simulink model "torqueBalancingPHRIStandup"  (Simulink 9.1)
settings: Solver=FixedStepDiscrete  StartTime=0.0  StopTime="Config.SIMULATION_TIME "  FixedStep=Config.Ts  RelTol=1e-3  EnableMultiTasking=on
InitFcn:
  | cd(fileparts(which(bdroot)));
  | initTorqueBalancingPHRIStandup;
StopFcn:
  | cd(fileparts(which(bdroot)));
  | stopTorqueBalancingPHRIStandup;
undefined symbols (not defined in the file or in its folder): bVectorConstraintsFeet, bVectorConstraintsLegs, Config, ConstraintsMatrixFeet, ConstraintsMatrixLegs, Gain, HUMAN_DOF_FOR_SIMULINK, Reg, ROBOT_DOF, ROBOT_DOF_FOR_SIMULINK, Sat, Sm
libraries: WBToolboxLibrary x153, simulink x4
(part 1 of 4)
settings Model: SuppressorTable=22 serialization::archive 11 0 6 0 0 0 1 0  Creator=daniele  LastModifiedBy=yeshi  NumberOfSteps=100
settings DataIOCC: LimitDataPoints=on
settings OptimizationCC: ExpressionDepthLimit=2147483647
settings DebuggingCC: SolverPrmCheckMsg=warning  FcnCallInpInsideContextMsg=warning  AllowSymbolicDim=off  StateNameClashWarn=warning
settings SFSimCC: SimParseCustomCode=off
settings GRTTargetCC: GeneratePreprocessorConditionals=Disable all

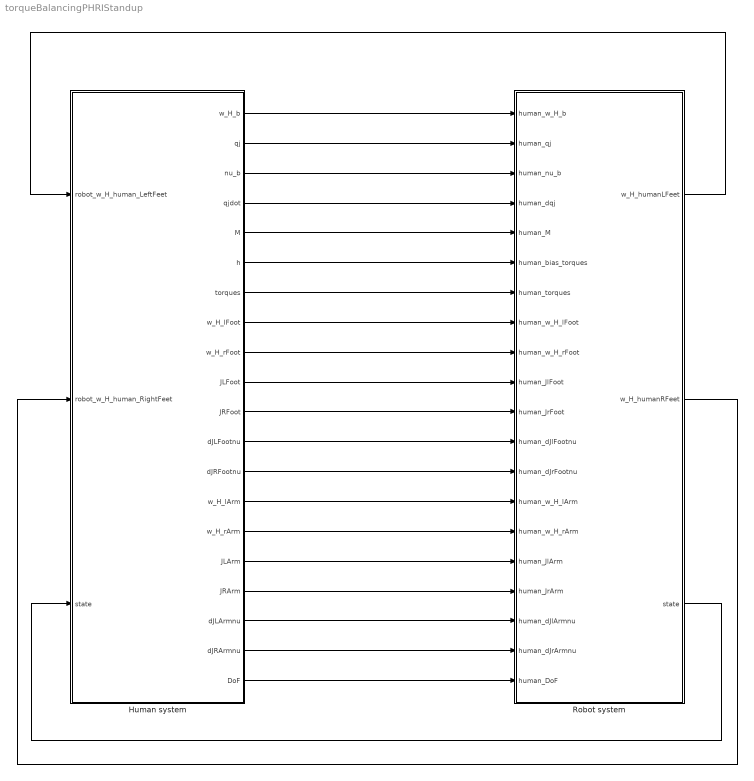
== system torqueBalancingPHRIStandup ==
  Human system : Subsystem
  Robot system : Subsystem
  wires:
  Human system/1(w_H_b) -> Robot system/1("human_w_H_b ")
  Human system/2(qj) -> Robot system/2("human_qj ")
  Human system/3(nu_b) -> Robot system/3(human_nu_b)
  Human system/4(qjdot) -> Robot system/4(human_dqj)
  Human system/5(M) -> Robot system/5(human_M)
  Human system/6(h) -> Robot system/6(human_bias_torques)
  Human system/7(torques) -> Robot system/7(human_torques)
  Human system/8(w_H_lFoot) -> Robot system/8(human_w_H_lFoot)
  Human system/9(w_H_rFoot) -> Robot system/9(human_w_H_rFoot)
  Human system/10(JLFoot) -> Robot system/10(human_JlFoot)
  Human system/11(JRFoot) -> Robot system/11(human_JrFoot)
  Human system/12(dJLFootnu) -> Robot system/12(human_dJlFootnu)
  Human system/13(dJRFootnu) -> Robot system/13(human_dJrFootnu)
  Human system/14(w_H_lArm) -> Robot system/14(human_w_H_lArm)
  Human system/15(w_H_rArm) -> Robot system/15(human_w_H_rArm)
  Human system/16(JLArm) -> Robot system/16(human_JlArm)
  Human system/17(JRArm) -> Robot system/17(human_JrArm)
  Human system/18(dJLArmnu) -> Robot system/18(human_dJlArmnu)
  Human system/19(dJRArmnu) -> Robot system/19(human_dJrArmnu)
  Human system/20(DoF) -> Robot system/20(human_DoF)
  Robot system/1(w_H_humanLFeet) -> Human system/1(robot_w_H_human_LeftFeet)
  Robot system/2(w_H_humanRFeet) -> Human system/2(robot_w_H_human_RightFeet)
  Robot system/3(state) -> Human system/3("state ")

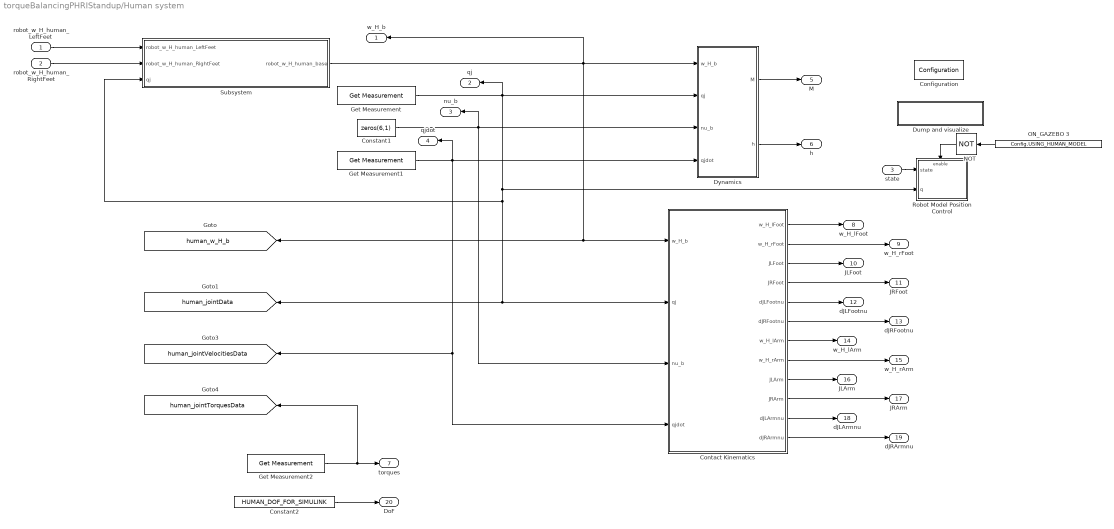
== system torqueBalancingPHRIStandup/Human system ==
  robot_w_H_human_LeftFeet : Inport
  robot_w_H_human_RightFeet : Inport  Port=2
  "state " : Inport  Port=3
  Configuration : WBToolboxLibrary/Utilities/Configuration  ConfigSource=Workspace  ConfigObject='HUMAN_WBTConfigRobot'  RobotName='icubSim'  UrdfFile='model.urdf'  ControlledJoints={'l_elbow','l_shoulder_pitch','torso_roll'}  ControlBoardsNames={'left_arm','right_arm','torso'}  LocalName='WBT'  GravityVector=[0,0,-9.81]
      settings: SourceProductName=Whole Body Toolbox
  Constant1 : Constant  Value=zeros(6,1)
  Constant2 : Constant  Value=HUMAN_DOF_FOR_SIMULINK
  Contact Kinematics : Subsystem
  Dump and visualize : Subsystem
      mask Display: disp('VISUALIZER')
  Dynamics : Subsystem
  Get Measurement : WBToolboxLibrary/wholeBodyStates/Get Measurement  measuredType=Joints Position
      settings: SourceProductName=Whole Body Toolbox
  Get Measurement1 : WBToolboxLibrary/wholeBodyStates/Get Measurement  measuredType=Joints Velocity
      settings: SourceProductName=Whole Body Toolbox
  Get Measurement2 : WBToolboxLibrary/wholeBodyStates/Get Measurement  measuredType=Joints Torque
      settings: SourceProductName=Whole Body Toolbox
  NOT : Logic  Operator=NOT  IconShape=distinctive  AllPortsSameDT=off  OutDataTypeStr=boolean
  ON_GAZEBO 3 : Constant  Value=Config.USING_HUMAN_MODEL
  Robot Model Position Control : Subsystem
  Subsystem : Subsystem
  w_H_b : Outport
  qj : Outport  Port=2
  nu_b : Outport  Port=3
  qjdot : Outport  Port=4
  M : Outport  Port=5
  h : Outport  Port=6
  torques : Outport  Port=7
  w_H_lFoot : Outport  Port=8
  w_H_rFoot : Outport  Port=9
  JLFoot : Outport  Port=10
  JRFoot : Outport  Port=11
  dJLFootnu : Outport  Port=12
  dJRFootnu : Outport  Port=13
  w_H_lArm : Outport  Port=14
  w_H_rArm : Outport  Port=15
  JLArm : Outport  Port=16
  JRArm : Outport  Port=17
  dJLArmnu : Outport  Port=18
  dJRArmnu : Outport  Port=19
  DoF : Outport  Port=20
  tag scope: human_jointData=global, human_jointTorquesData=global, human_jointVelocitiesData=global, human_w_H_b=global
  wires:
  Constant1/1 -> nu_b/1, Contact Kinematics/3(nu_b), Dynamics/3(nu_b)
  Get Measurement1/1 -> qjdot/1, Dynamics/4(qjdot), [human_jointVelocitiesData], Contact Kinematics/4(qjdot)
  Dynamics/1(M) -> M/1
  Dynamics/2(h) -> h/1
  Get Measurement2/1 -> [human_jointTorquesData], torques/1
  Contact Kinematics/1(w_H_lFoot) -> w_H_lFoot/1
  Contact Kinematics/2(w_H_rFoot) -> w_H_rFoot/1
  Contact Kinematics/3(JLFoot) -> JLFoot/1
  Contact Kinematics/4(JRFoot) -> JRFoot/1
  Contact Kinematics/5(dJLFootnu) -> dJLFootnu/1
  Contact Kinematics/6(dJRFootnu) -> dJRFootnu/1
  Contact Kinematics/7(w_H_lArm) -> w_H_lArm/1
  Contact Kinematics/8(w_H_rArm) -> w_H_rArm/1
  Contact Kinematics/9(JLArm) -> JLArm/1
  Contact Kinematics/10(JRArm) -> JRArm/1
  Contact Kinematics/11(dJLArmnu) -> dJLArmnu/1
  Contact Kinematics/12(dJRArmnu) -> dJRArmnu/1
  Constant2/1 -> DoF/1
  Get Measurement/1 -> qj/1, [human_jointData], Contact Kinematics/2(qj), Subsystem/3(qj), Robot Model Position Control/2(q), Dynamics/2(qj)
  Subsystem/1(robot_w_H_human_base) -> w_H_b/1, Contact Kinematics/1(w_H_b), [human_w_H_b], Dynamics/1(w_H_b)
  robot_w_H_human_LeftFeet/1 -> Subsystem/1(robot_w_H_human_LeftFeet)
  robot_w_H_human_RightFeet/1 -> Subsystem/2(robot_w_H_human_RightFeet)
  "state "/1 -> Robot Model Position Control/1(state)
  ON_GAZEBO 3/1 -> NOT/1
  NOT/1 -> Robot Model Position Control/Enable

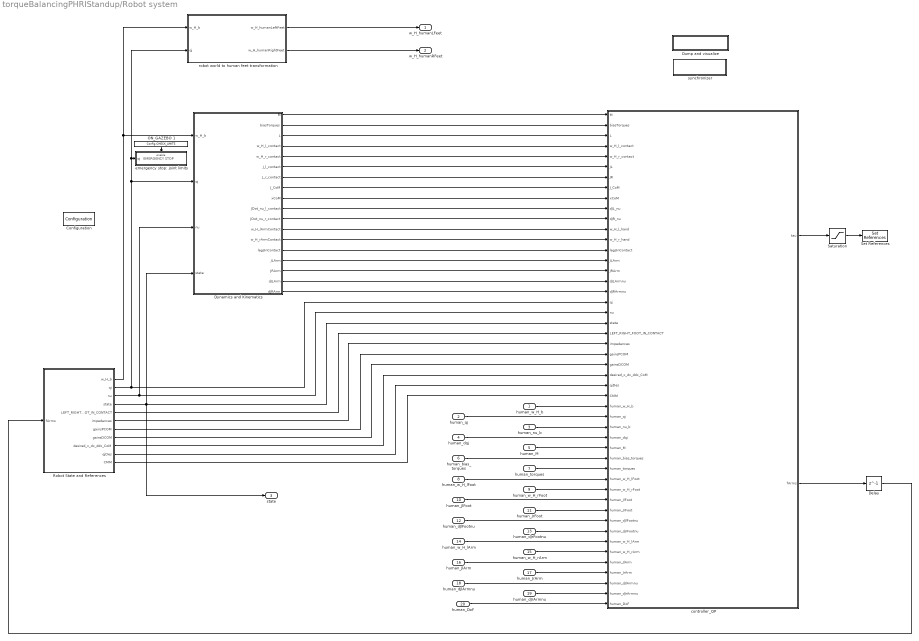
== system torqueBalancingPHRIStandup/Robot system ==
  "human_w_H_b " : Inport
  "human_qj " : Inport  Port=2
  human_nu_b : Inport  Port=3
  human_dqj : Inport  Port=4
  human_M : Inport  Port=5
  human_bias_torques : Inport  Port=6
  human_torques : Inport  Port=7
  human_w_H_lFoot : Inport  Port=8
  human_w_H_rFoot : Inport  Port=9
  human_JlFoot : Inport  Port=10
  human_JrFoot : Inport  Port=11
  human_dJlFootnu : Inport  Port=12
  human_dJrFootnu : Inport  Port=13
  human_w_H_lArm : Inport  Port=14
  human_w_H_rArm : Inport  Port=15
  human_JlArm : Inport  Port=16
  human_JrArm : Inport  Port=17
  human_dJlArmnu : Inport  Port=18
  human_dJrArmnu : Inport  Port=19
  human_DoF : Inport  Port=20
  Configuration : WBToolboxLibrary/Utilities/Configuration  ConfigSource=Workspace  ConfigObject='WBTConfigRobot'  RobotName='icubSim'  UrdfFile='model.urdf'  ControlledJoints={'l_elbow','l_shoulder_pitch','torso_roll'}  ControlBoardsNames={'left_arm','right_arm','torso'}  LocalName='WBT'  GravityVector=[0,0,-9.81]
      settings: SourceProductName=Whole Body Toolbox
  Delay : Delay  DelayLength=1
  Dump and visualize : Subsystem
      mask Display: disp('VISUALIZER')
  Dynamics and Kinematics : Subsystem
  ON_GAZEBO 1 : Constant  Value=Config.CHECK_LIMITS
  Robot State and References : Subsystem  Priority=-10
  Saturation : Saturate  UpperLimit=Sat.torque  LowerLimit=-Sat.torque
  Set References : WBToolboxLibrary/wholeBodyActuators/Set References  controlType=Torque  refSpeed=50  refAcceleration=1000000*(pi/180)
      settings: SourceProductName=Whole Body Toolbox
  controller_QP : Subsystem
  emergency stop: joint limits : Subsystem
  robot world to human feet transformation : Subsystem
  synchronizer : Subsystem
      mask Display: disp('SYNCHRONIZER')
  w_H_humanLFeet : Outport
  w_H_humanRFeet : Outport  Port=2
  state : Outport  Port=3
  wires:
  Dynamics and Kinematics/9(xCoM) -> controller_QP/9(xCoM)
  Saturation/1 -> Set References/1
  Robot State and References/6(impedances) -> controller_QP/23(impedances)
  Robot State and References/7(gainsPCOM) -> controller_QP/24(gainsPCOM)
  Dynamics and Kinematics/10(JDot_nu_l_contact) -> controller_QP/10(dJL_nu)
  Robot State and References/5(LEFT_RIGHT_FOOT_IN_CONTACT) -> controller_QP/22(LEFT_RIGHT_FOOT_IN_CONTACT)
  Dynamics and Kinematics/2(biasTorques) -> controller_QP/2(biasTorques)
  ON_GAZEBO 1/1 -> emergency stop: joint limits/Enable
  Dynamics and Kinematics/6(J_l_contact) -> controller_QP/6(JL)
  Dynamics and Kinematics/14(legsInContact) -> controller_QP/14(legsInContact)
  Dynamics and Kinematics/8(J_CoM) -> controller_QP/8(J_CoM)
  Robot State and References/4(state) -> state/1, Dynamics and Kinematics/4("state "), controller_QP/21(state)
  Dynamics and Kinematics/4(w_H_l_contact) -> controller_QP/4(w_H_l_contact)
  Robot State and References/2(qj) -> robot world to human feet transformation/2(qj), emergency stop: joint limits/1(qj   EMERGENCY STOP), Dynamics and Kinematics/2(qj), controller_QP/19(qj)
  Dynamics and Kinematics/11(JDot_nu_r_contact) -> controller_QP/11(dJR_nu)
  Robot State and References/10(qjDes) -> controller_QP/27(qjDes)
  Robot State and References/9(desired_x_dx_ddx_CoM) -> controller_QP/26(desired_x_dx_ddx_CoM)
  Dynamics and Kinematics/1(M) -> controller_QP/1(M)
  Dynamics and Kinematics/5(w_H_r_contact) -> controller_QP/5(w_H_r_contact)
  Robot State and References/8(gainsDCOM) -> controller_QP/25(gainsDCOM)
  Robot State and References/1(w_H_b) -> robot world to human feet transformation/1(w_H_b), Dynamics and Kinematics/1(w_H_b)
  Robot State and References/3(nu) -> Dynamics and Kinematics/3(nu), controller_QP/20(nu)
  controller_QP/1("tau ") -> Saturation/1
  Dynamics and Kinematics/7(J_r_contact) -> controller_QP/7(JR)
  Dynamics and Kinematics/3(L) -> controller_QP/3("L ")
  robot world to human feet transformation/2(w_H_humanRightFeet) -> w_H_humanRFeet/1
  robot world to human feet transformation/1(w_H_humanLeftFeet) -> w_H_humanLFeet/1
  "human_w_H_b "/1 -> controller_QP/29("human_w_H_b ")
  "human_qj "/1 -> controller_QP/30("human_qj ")
  human_nu_b/1 -> controller_QP/31(human_nu_b)
  human_dqj/1 -> controller_QP/32(human_dqj)
  human_M/1 -> controller_QP/33(human_M)
  human_bias_torques/1 -> controller_QP/34(human_bias_torques)
  human_torques/1 -> controller_QP/35(human_torques)
  human_w_H_lFoot/1 -> controller_QP/36(human_w_H_lFoot)
  human_w_H_rFoot/1 -> controller_QP/37(human_w_H_rFoot)
  human_JlFoot/1 -> controller_QP/38(human_JlFoot)
  human_JrFoot/1 -> controller_QP/39(human_JrFoot)
  human_dJlFootnu/1 -> controller_QP/40(human_dJlFootnu)
  human_dJrFootnu/1 -> controller_QP/41(human_dJrFootnu)
  human_w_H_lArm/1 -> controller_QP/42(human_w_H_lArm)
  human_w_H_rArm/1 -> controller_QP/43(human_w_H_rArm)
  human_JlArm/1 -> controller_QP/44(human_JlArm)
  human_JrArm/1 -> controller_QP/45(human_JrArm)
  human_dJlArmnu/1 -> controller_QP/46(human_dJlArmnu)
  human_dJrArmnu/1 -> controller_QP/47(human_dJrArmnu)
  human_DoF/1 -> controller_QP/48(human_DoF)
  Dynamics and Kinematics/12(w_H_lArmContact) -> controller_QP/12(w_H_l_hand)
  Dynamics and Kinematics/13(w_H_rArmContact) -> controller_QP/13(w_H_r_hand)
  Dynamics and Kinematics/15(JLArm) -> controller_QP/15(JLArm)
  Dynamics and Kinematics/16(JRArm) -> controller_QP/16(JRArm)
  Dynamics and Kinematics/17(dJLArm) -> controller_QP/17(dJLArmnu)
  Dynamics and Kinematics/18(dJRArm) -> controller_QP/18(dJRArmnu)
  controller_QP/2(fArms) -> Delay/1
  Delay/1 -> Robot State and References/1(fArms)
  Robot State and References/11(CMM) -> controller_QP/28(CMM)

== system torqueBalancingPHRIStandup/Human system/Contact Kinematics ==
  w_H_b : Inport
  qj : Inport  Port=2
  nu_b : Inport  Port=3
  qjdot : Inport  Port=4
  Arm Contact Kinematics : Subsystem
  Leg Contact Kinematics : Subsystem
  w_H_lFoot : Outport
  w_H_rFoot : Outport  Port=2
  JLFoot : Outport  Port=3
  JRFoot : Outport  Port=4
  dJLFootnu : Outport  Port=5
  dJRFootnu : Outport  Port=6
  w_H_lArm : Outport  Port=7
  w_H_rArm : Outport  Port=8
  JLArm : Outport  Port=9
  JRArm : Outport  Port=10
  dJLArmnu : Outport  Port=11
  dJRArmnu : Outport  Port=12
  wires:
  w_H_b/1 -> Arm Contact Kinematics/1(w_H_b), Leg Contact Kinematics/1(w_H_b)
  qj/1 -> Arm Contact Kinematics/2(qj), Leg Contact Kinematics/2(qj)
  nu_b/1 -> Leg Contact Kinematics/3(nu_b), Arm Contact Kinematics/3(nu_b)
  qjdot/1 -> Arm Contact Kinematics/4(qjdot), Leg Contact Kinematics/4(qjdot)
  Leg Contact Kinematics/1(w_H_lFoot) -> w_H_lFoot/1
  Leg Contact Kinematics/2(w_H_rFoot) -> w_H_rFoot/1
  Leg Contact Kinematics/3(JLFoot) -> JLFoot/1
  Leg Contact Kinematics/4(JRFoot) -> JRFoot/1
  Leg Contact Kinematics/5(dJLFootnu) -> dJLFootnu/1
  Leg Contact Kinematics/6(dJRFootnu) -> dJRFootnu/1
  Arm Contact Kinematics/2(w_H_rArm) -> w_H_rArm/1
  Arm Contact Kinematics/1(w_H_lArm) -> w_H_lArm/1
  Arm Contact Kinematics/3(JLArm) -> JLArm/1
  Arm Contact Kinematics/5(dJLArmnu) -> dJLArmnu/1
  Arm Contact Kinematics/6(dJRArmnu) -> dJRArmnu/1
  Arm Contact Kinematics/4(JRArm) -> JRArm/1

== system torqueBalancingPHRIStandup/Human system/Dump and visualize ==
  Human data : Subsystem
  Logical Operator1 : Logic  Operator=OR  AllPortsSameDT=off  OutDataTypeStr=boolean
  ON_GAZEBO 3 : Constant  Value=Config.SCOPES_ALL
  ON_GAZEBO 4 : Constant  Value=Config.SCOPES_MAIN
  wires:
  ON_GAZEBO 3/1 -> Logical Operator1/1
  ON_GAZEBO 4/1 -> Logical Operator1/2
  Logical Operator1/1 -> Human data/Enable
  [human_jointVelocitiesData] -> Human data/3(human_jointVelocitiesData)
  [human_jointTorquesData] -> Human data/4(human_jointTorquesData)
  [human_w_H_b] -> Human data/1(human_w_H_b)
  [human_jointData] -> Human data/2(human_jointData)

== system torqueBalancingPHRIStandup/Human system/Dynamics ==
  w_H_b : Inport
  qj : Inport  Port=2
  nu_b : Inport  Port=3
  qjdot : Inport  Port=4
  Get Bias Forces : WBToolboxLibrary/wholeBodyModel/Dynamics/Get Bias Forces
      settings: SourceProductName=Whole Body Toolbox
  Mass Matrix : WBToolboxLibrary/wholeBodyModel/Dynamics/Mass Matrix
      settings: SourceProductName=Whole Body Toolbox
  M : Outport
  h : Outport  Port=2
  wires:
  qjdot/1 -> Get Bias Forces/4
  nu_b/1 -> Get Bias Forces/3
  qj/1 -> Get Bias Forces/2, Mass Matrix/2
  Get Bias Forces/1 -> h/1
  w_H_b/1 -> Get Bias Forces/1, Mass Matrix/1
  Mass Matrix/1 -> M/1

== system torqueBalancingPHRIStandup/Human system/Robot Model Position Control ==
  state : Inport
  q : Inport  Port=2
  Enable : EnablePort
  Clock : Clock
  Constant : Constant  Value=2
  Demux1 : Demux  Outputs=Config.numOfJointsForEachControlboard
  Minimum Jerk Trajectory Generator1 : WBToolboxLibrary/Utilities/Minimum Jerk Trajectory Generator  externalSettlingTime=on  settlingTime=1  sampleTime=Config.Ts  resetOnSettlingTime=off  firstDerivatives=off  secondDerivatives=off  explicitInitialValue=off
      settings: SourceProductName=Whole Body Toolbox
  Set References : WBToolboxLibrary/wholeBodyActuators/Set References  controlType=Position Direct  refSpeed=2*(pi/180)  refAcceleration=1000000*(pi/180)
      settings: SourceProductName=Whole Body Toolbox
  getJointRef : MATLAB Function  TreatAsAtomicUnit=on
  joint references : Scope  NumInputPorts=6
  wires:
  getJointRef/1(joint_ref) -> Minimum Jerk Trajectory Generator1/1
  Constant/1 -> Minimum Jerk Trajectory Generator1/2
  Demux1/3 -> joint references/3  "right_arm"
  Demux1/5 -> joint references/5  "right_leg"
  Demux1/4 -> joint references/4  "left_leg"
  Demux1/2 -> joint references/2  "left_arm"
  Minimum Jerk Trajectory Generator1/1 -> Demux1/1, Set References/1
  state/1 -> getJointRef/3(state), joint references/6
  Demux1/1 -> joint references/1  "torso"
  Clock/1 -> getJointRef/1(sim_time)
  q/1 -> getJointRef/2(q)

== system torqueBalancingPHRIStandup/Human system/Subsystem ==
  robot_w_H_human_LeftFeet : Inport
  robot_w_H_human_RightFeet : Inport  Port=2
  qj : Inport  Port=3
  Constant3 : Constant  Value=eye(4)
  Forward Kinematics : WBToolboxLibrary/wholeBodyModel/Kinematics/Forward Kinematics  frameName=HUMAN_Frames.LEFT_FOOT
      settings: SourceProductName=Whole Body Toolbox
  "Inv\\*  " : Product  Inputs=*/  Multiplication=Matrix(*)
  Switch : Switch  Criteria=u2 > Threshold
  switch threshold : Constant
  robot_w_H_human_base : Outport
  wires:
  robot_w_H_human_RightFeet/1 -> Switch/3
  "Inv\\*  "/1 -> robot_w_H_human_base/1
  qj/1 -> Forward Kinematics/2
  switch threshold/1 -> Switch/2
  Constant3/1 -> Forward Kinematics/1
  Switch/1 -> "Inv\\*  "/1
  Forward Kinematics/1 -> "Inv\\*  "/2
  robot_w_H_human_LeftFeet/1 -> Switch/1

== system torqueBalancingPHRIStandup/Robot system/Dump and visualize ==
  Human assistance : Subsystem
  Logical Operator2 : Logic  Operator=OR  AllPortsSameDT=off  OutDataTypeStr=boolean
  ON_GAZEBO 1 : Constant  Value=Config.SCOPES_ALL
  ON_GAZEBO 2 : Constant  Value=Config.SCOPES_MAIN
  Robot data1 : Subsystem
  wires:
  [alpha] -> Human assistance/2(alpha)
  [fArms] -> Human assistance/3(fArms)
  [phri_human_feet_wrench] -> Human assistance/4(phri_human_feet_wrench)
  [phri_robot_feet_wrench] -> Human assistance/5(phri_robot_feet_wrench)
  [f_noQP] -> Robot data1/8(fDesNoQP)
  ON_GAZEBO 2/1 -> Logical Operator2/2
  [CoM_error] -> Robot data1/5(CoM_Error)
  [state] -> Human assistance/1(state), Robot data1/3(state)
  [qj_des] -> Robot data1/4(qj_des)
  [CoM_des] -> Robot data1/7(CoM_des)
  [w_H_b] -> Robot data1/2(w_H_b)
  Logical Operator2/1 -> Robot data1/Enable
  ON_GAZEBO 1/1 -> Logical Operator2/1
  [tau_des] -> Robot data1/1(tau_des)
  [f_QP] -> Robot data1/6(fDesQP)

== system torqueBalancingPHRIStandup/Robot system/Dynamics and Kinematics ==
  w_H_b : Inport
  qj : Inport  Port=2
  nu : Inport  Port=3
  "state " : Inport  Port=4
  Dynamics : Subsystem
  Kinematics : Subsystem
  M : Outport
  biasTorques : Outport  Port=2
  L : Outport  Port=3
  w_H_l_contact : Outport  Port=4
  w_H_r_contact : Outport  Port=5
  J_l_contact : Outport  Port=6
  J_r_contact : Outport  Port=7
  J_CoM : Outport  Port=8
  xCoM : Outport  Port=9
  JDot_nu_l_contact : Outport  Port=10
  JDot_nu_r_contact : Outport  Port=11
  w_H_lArmContact : Outport  Port=12
  w_H_rArmContact : Outport  Port=13
  legsInContact : Outport  Port=14
  JLArm : Outport  Port=15
  JRArm : Outport  Port=16
  dJLArm : Outport  Port=17
  dJRArm : Outport  Port=18
  wires:
  w_H_b/1 -> Kinematics/3(w_H_b), Dynamics/1(w_H_b)
  qj/1 -> Dynamics/2(qj), Kinematics/2(qj)
  nu/1 -> Dynamics/3(nu), Kinematics/1(nu)
  Dynamics/1(M(q)) -> M/1
  Dynamics/2(biasTorques) -> biasTorques/1
  Dynamics/3(L(q,dq)) -> L/1
  Kinematics/5(J_CoM) -> J_CoM/1
  Kinematics/6(xCoM) -> xCoM/1
  Kinematics/1(w_H_l_contact) -> w_H_l_contact/1
  Kinematics/2(w_H_r_contact) -> w_H_r_contact/1
  Kinematics/7(JDot_nu_l_contact) -> JDot_nu_l_contact/1
  Kinematics/8(JDot_nu_r_contact) -> JDot_nu_r_contact/1
  Kinematics/3(J_l_contact) -> J_l_contact/1
  Kinematics/4(J_r_contact) -> J_r_contact/1
  Kinematics/9(legsInContact) -> legsInContact/1
  "state "/1 -> Kinematics/4("state ")
  Kinematics/12(JLArm) -> JLArm/1
  Kinematics/11(w_H_rArmContact) -> w_H_rArmContact/1
  Kinematics/13(JRArm) -> JRArm/1
  Kinematics/15(JDot_nu_rArm_contact) -> dJRArm/1
  Kinematics/14(JDot_nu_lArm_contact) -> dJLArm/1
  Kinematics/10(w_H_lArmContact) -> w_H_lArmContact/1

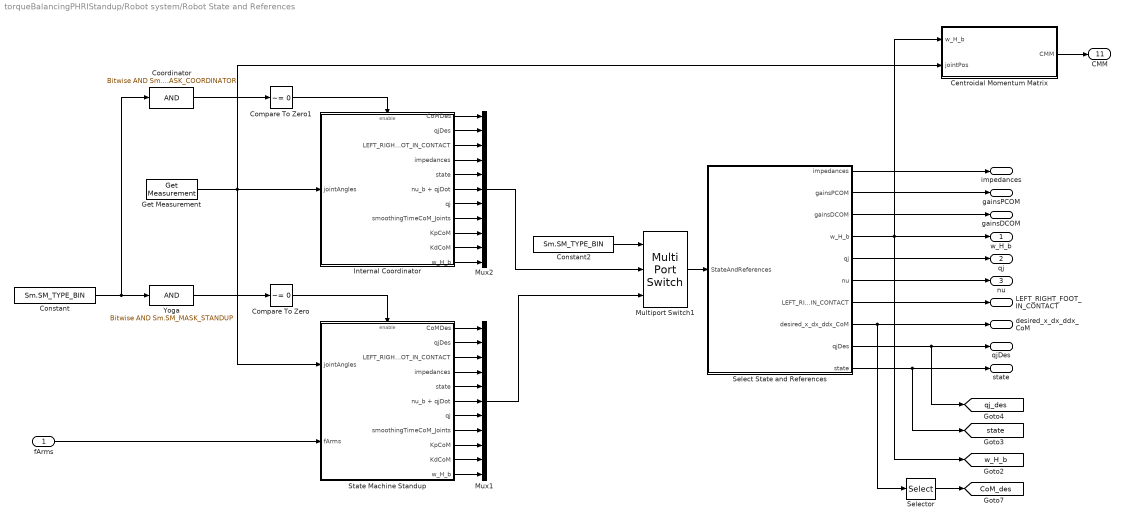
== system torqueBalancingPHRIStandup/Robot system/Robot State and References ==
  fArms : Inport
  "Centroidal Momentum Matrix " : Subsystem
  Compare To Zero : simulink/Logic and Bit Operations/Compare To Zero  relop=~=  OutDataTypeStr=boolean
  Compare To Zero1 : simulink/Logic and Bit Operations/Compare To Zero  relop=~=  OutDataTypeStr=boolean
  Constant : Constant  Priority=-10  Value=Sm.SM_TYPE_BIN  OutDataTypeStr=uint8
  Constant2 : Constant  Priority=-10  Value=Sm.SM_TYPE_BIN  OutDataTypeStr=uint8
  Coordinator : simulink/Logic and Bit Operations/Bitwise Operator  logicop=AND  UseBitMask=on  BitMask=Sm.SM_MASK_COORDINATOR  BitMaskRealWorld=Stored Integer
  Get Measurement : WBToolboxLibrary/wholeBodyStates/Get Measurement  measuredType=Joints Position
      settings: SourceProductName=Whole Body Toolbox
  Internal Coordinator : Subsystem
  Multiport Switch1 : MultiPortSwitch  DataPortOrder=Specify indices  DataPortIndices={1, 2}
  Mux1 : Mux  Inputs=11
  Mux2 : Mux  Inputs=11
  Select State and References : Subsystem
  Selector : Selector  NumberOfDimensions=2  InputPortWidth=3  IndexOptions=Index vector (dialog),Index vector (dialog)  Indices=[1 2 3],[1]  OutputSizes=1,1
  State Machine Standup : Subsystem  Priority=-100
  Yoga : simulink/Logic and Bit Operations/Bitwise Operator  logicop=AND  UseBitMask=on  BitMask=Sm.SM_MASK_STANDUP  BitMaskRealWorld=Stored Integer
  w_H_b : Outport
  qj : Outport  Port=2
  nu : Outport  Port=3
  state : Outport  Port=4
  LEFT_RIGHT_FOOT_IN_CONTACT : Outport  Port=5
  impedances : Outport  Port=6
  gainsPCOM : Outport  Port=7
  gainsDCOM : Outport  Port=8
  desired_x_dx_ddx_CoM : Outport  Port=9
  qjDes : Outport  Port=10
  CMM : Outport  Port=11
  tag scope: CoM_des=global, qj_des=global, state=global, w_H_b=global
  wires:
  Constant/1 -> Yoga/1, Coordinator/1
  State Machine Standup/3(LEFT_RIGHT_FOOT_IN_CONTACT) -> Mux1/3
  State Machine Standup/2(qjDes) -> Mux1/2
  State Machine Standup/1(CoMDes) -> Mux1/1
  Internal Coordinator/1(CoMDes) -> Mux2/1
  Internal Coordinator/2(qjDes) -> Mux2/2
  Internal Coordinator/3(LEFT_RIGHT_FOOT_IN_CONTACT) -> Mux2/3
  State Machine Standup/4(impedances) -> Mux1/4
  Internal Coordinator/4(impedances) -> Mux2/4
  State Machine Standup/5(state) -> Mux1/5
  Internal Coordinator/5(state) -> Mux2/5
  Internal Coordinator/6(nu_b + qjDot) -> Mux2/6
  Internal Coordinator/7(qj) -> Mux2/7
  State Machine Standup/6(nu_b + qjDot) -> Mux1/6
  State Machine Standup/7(qj) -> Mux1/7
  Coordinator/1 -> Compare To Zero1/1
  Yoga/1 -> Compare To Zero/1
  Compare To Zero/1 -> State Machine Standup/Enable
  Compare To Zero1/1 -> Internal Coordinator/Enable
  Internal Coordinator/8(smoothingTimeCoM_Joints) -> Mux2/8
  State Machine Standup/8(smoothingTimeCoM_Joints) -> Mux1/8
  State Machine Standup/9(KpCoM) -> Mux1/9
  State Machine Standup/10(KdCoM) -> Mux1/10
  Internal Coordinator/9(KpCoM) -> Mux2/9
  Internal Coordinator/10(KdCoM) -> Mux2/10
  Constant2/1 -> Multiport Switch1/1
  Get Measurement/1 -> "Centroidal Momentum Matrix "/2(jointPos), Internal Coordinator/1(jointAngles), State Machine Standup/1(jointAngles)
  State Machine Standup/11(w_H_b) -> Mux1/11
  Internal Coordinator/11(w_H_b) -> Mux2/11
  Mux2/1 -> Multiport Switch1/2
  Multiport Switch1/1 -> Select State and References/1(StateAndReferences)
  Select State and References/1(impedances) -> impedances/1
  Select State and References/2(gainsPCOM) -> gainsPCOM/1
  Select State and References/3(gainsDCOM) -> gainsDCOM/1
  Select State and References/4(w_H_b) -> "Centroidal Momentum Matrix "/1(w_H_b), w_H_b/1, [w_H_b]
  Select State and References/5(qj) -> qj/1
  Select State and References/6(nu) -> nu/1
  Select State and References/7(LEFT_RIGHT_FOOT_IN_CONTACT) -> LEFT_RIGHT_FOOT_IN_CONTACT/1
  Select State and References/8(desired_x_dx_ddx_CoM) -> desired_x_dx_ddx_CoM/1, Selector/1
  Select State and References/9(qjDes) -> qjDes/1, [qj_des]
  Select State and References/10(state) -> state/1, [state]
  Selector/1 -> [CoM_des]
  Mux1/1 -> Multiport Switch1/3
  fArms/1 -> State Machine Standup/2(fArms)
  "Centroidal Momentum Matrix "/1(CMM) -> CMM/1

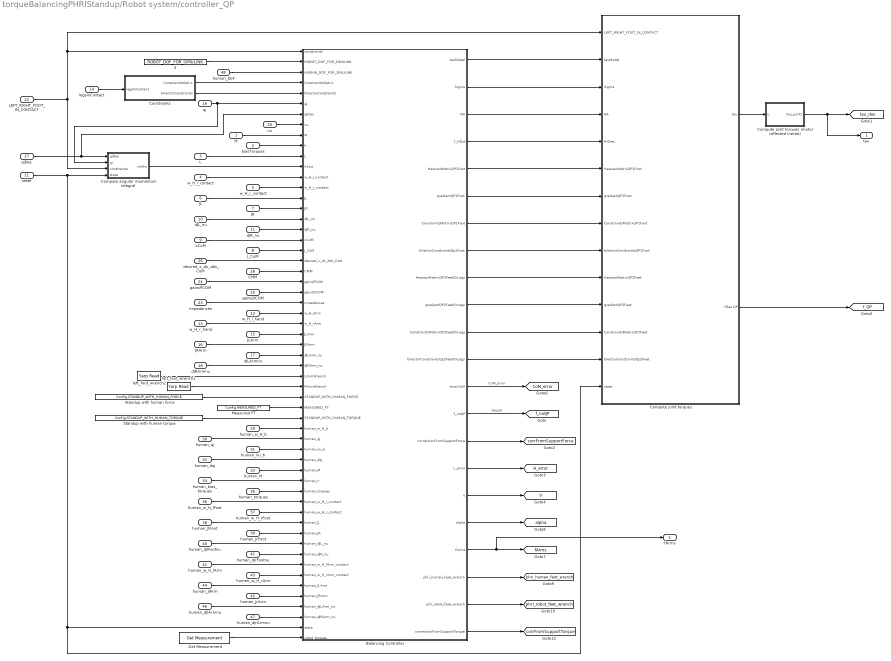
== system torqueBalancingPHRIStandup/Robot system/controller_QP ==
  M : Inport
  biasTorques : Inport  Port=2
  "L " : Inport  Port=3
  w_H_l_contact : Inport  Port=4
  w_H_r_contact : Inport  Port=5
  JL : Inport  Port=6
  JR : Inport  Port=7
  J_CoM : Inport  Port=8
  xCoM : Inport  Port=9
  dJL_nu : Inport  Port=10
  dJR_nu : Inport  Port=11
  w_H_l_hand : Inport  Port=12
  w_H_r_hand : Inport  Port=13
  legsInContact : Inport  Port=14
  JLArm : Inport  Port=15
  JRArm : Inport  Port=16
  dJLArmnu : Inport  Port=17
  dJRArmnu : Inport  Port=18
  qj : Inport  Port=19
  nu : Inport  Port=20
  state : Inport  Port=21
  LEFT_RIGHT_FOOT_IN_CONTACT : Inport  Port=22
  impedances : Inport  Port=23
  gainsPCOM : Inport  Port=24
  gainsDCOM : Inport  Port=25
  desired_x_dx_ddx_CoM : Inport  Port=26
  qjDes : Inport  Port=27
  CMM : Inport  Port=28
  "human_w_H_b " : Inport  Port=29
  "human_qj " : Inport  Port=30
  human_nu_b : Inport  Port=31
  human_dqj : Inport  Port=32
  human_M : Inport  Port=33
  human_bias_torques : Inport  Port=34
  human_torques : Inport  Port=35
  human_w_H_lFoot : Inport  Port=36
  human_w_H_rFoot : Inport  Port=37
  human_JlFoot : Inport  Port=38
  human_JrFoot : Inport  Port=39
  human_dJlFootnu : Inport  Port=40
  human_dJrFootnu : Inport  Port=41
  human_w_H_lArm : Inport  Port=42
  human_w_H_rArm : Inport  Port=43
  human_JlArm : Inport  Port=44
  human_JrArm : Inport  Port=45
  human_dJlArmnu : Inport  Port=46
  human_dJrArmnu : Inport  Port=47
  human_DoF : Inport  Port=48
  "    5" : Constant  Value=ROBOT_DOF_FOR_SIMULINK
  "Balancing Controller " : MATLAB Function  TreatAsAtomicUnit=on
  Compute angular momentum integral : Subsystem
  Compute joint torques : Subsystem
  Compute joint torques (motor reflected inertia) : Subsystem
  Constraints : Subsystem
  Get Measurement : WBToolboxLibrary/wholeBodyStates/Get Measurement  measuredType=Joints Torque
      settings: SourceProductName=Whole Body Toolbox
  Measured FT : Constant  Value=Config.MEASURED_FT
  Standup with human force : Constant  Value=Config.STANDUP_WITH_HUMAN_FORCE
  Standup with human torque : Constant  Value=Config.STANDUP_WITH_HUMAN_TORQUE
  left_foot_wrench1 : WBToolboxLibrary/Utilities/Yarp Read  portName=Ports.RIGHT_ARM  signalSize=6  timeout=0.5  blocking=off  timestamp=off  autoconnect=on  errorOnConnection=on
      settings: SourceProductName=Whole Body Toolbox
  left_foot_wrench2 : WBToolboxLibrary/Utilities/Yarp Read  portName=Ports.LEFT_ARM  signalSize=6  timeout=0.5  blocking=off  timestamp=off  autoconnect=on  errorOnConnection=on
      settings: SourceProductName=Whole Body Toolbox
  "tau " : Outport
  fArms : Outport  Port=2
  tag scope: CoM_error=global, H_error=global, V=global, alpha=global, corrFromSupportForce=global, corrFromSupportTorque=global, fArms=global, f_QP=global, f_noQP=global, phri_human_feet_wrench=global, phri_robot_feet_wrench=global, tau_des=global
  wires:
  LEFT_RIGHT_FOOT_IN_CONTACT/1 -> Compute joint torques/1(LEFT_RIGHT_FOOT_IN_CONTACT), "Balancing Controller "/1(constraints), Compute angular momentum integral/3(constraints)
  qj/1 -> "Balancing Controller "/6(qj), Compute angular momentum integral/2(qj)
  qjDes/1 -> "Balancing Controller "/7(qjDes), Compute angular momentum integral/1(qjDes)
  M/1 -> "Balancing Controller "/9(M)
  biasTorques/1 -> "Balancing Controller "/10(h)
  desired_x_dx_ddx_CoM/1 -> "Balancing Controller "/21(desired_x_dx_ddx_CoM)
  impedances/1 -> "Balancing Controller "/25(impedances)
  "L "/1 -> "Balancing Controller "/11(L)
  "    5"/1 -> "Balancing Controller "/2(ROBOT_DOF_FOR_SIMULINK)
  Constraints/1(ConstraintsMatrix) -> "Balancing Controller "/4(ConstraintsMatrix)
  Constraints/2(bVectorConstraints) -> "Balancing Controller "/5(bVectorConstraints)
  nu/1 -> "Balancing Controller "/8(nu)
  gainsPCOM/1 -> "Balancing Controller "/23(gainsPCOM)
  gainsDCOM/1 -> "Balancing Controller "/24(gainsDCOM)
  w_H_r_contact/1 -> "Balancing Controller "/14(w_H_r_contact)
  w_H_l_contact/1 -> "Balancing Controller "/13(w_H_l_contact)
  JL/1 -> "Balancing Controller "/15(JL)
  JR/1 -> "Balancing Controller "/16(JR)
  Compute angular momentum integral/1(intHw) -> "Balancing Controller "/12(intLw)
  dJL_nu/1 -> "Balancing Controller "/17(dJL_nu)
  dJR_nu/1 -> "Balancing Controller "/18(dJR_nu)
  J_CoM/1 -> "Balancing Controller "/20(J_CoM)
  xCoM/1 -> "Balancing Controller "/19(xCoM)
  state/1 -> Compute joint torques/14(state), "Balancing Controller "/56(state), Compute angular momentum integral/4(state)
  Compute joint torques/1("tau ") -> Compute joint torques (motor reflected inertia)/1(u)
  "Balancing Controller "/1(tauModel) -> Compute joint torques/2(tauModel)
  "Balancing Controller "/2(Sigma) -> Compute joint torques/3(Sigma)
  "Balancing Controller "/3(NA) -> Compute joint torques/4(NA)
  "Balancing Controller "/4(f_HDot) -> Compute joint torques/5(fHDes)
  "Balancing Controller "/5(HessianMatrixQP1Foot) -> Compute joint torques/6(HessianMatrixQP1Foot)
  "Balancing Controller "/6(gradientQP1Foot) -> Compute joint torques/7(gradientQP1Foot)
  "Balancing Controller "/7(ConstraintsMatrixQP1Foot) -> Compute joint torques/8(ConstraintsMatrixQP1Foot)
  "Balancing Controller "/8(bVectorConstraintsQp1Foot) -> Compute joint torques/9(bVectorConstraintsQP1Foot)
  "Balancing Controller "/9(HessianMatrixQP2FeetOrLegs) -> Compute joint torques/10(HessianMatrixQP2Feet)
  "Balancing Controller "/10(gradientQP2FeetOrLegs) -> Compute joint torques/11(gradientQP2Feet)
  "Balancing Controller "/11(ConstraintsMatrixQP2FeetOrLegs) -> Compute joint torques/12(ConstraintsMatrixQP2Feet)
  "Balancing Controller "/12(bVectorConstraintsQp2FeetOrLegs) -> Compute joint torques/13(bVectorConstraintsQp2Feet)
  "Balancing Controller "/13(errorCoM) -> [CoM_error]  "CoM_Error"
  Compute joint torques/2(fDes QP) -> [f_QP]
  "Balancing Controller "/14(f_noQP) -> [f_noQP]  "fNoQP"
  Standup with human force/1 -> "Balancing Controller "/34(STANDUP_WITH_HUMAN_FORCE)
  left_foot_wrench2/1 -> "Balancing Controller "/32(LArmWrench)
  left_foot_wrench1/1 -> "Balancing Controller "/33(RArmWrench)
  w_H_l_hand/1 -> "Balancing Controller "/26(w_H_lArm)
  w_H_r_hand/1 -> "Balancing Controller "/27(w_H_rArm)
  legsInContact/1 -> Constraints/1(legsInContact)
  "Balancing Controller "/17(V) -> [V]
  "Balancing Controller "/16(L_error) -> [H_error]
  "Balancing Controller "/15(correctionFromSupportForce) -> [corrFromSupportForce]
  Compute joint torques (motor reflected inertia)/1(tau_joints) -> "tau "/1, [tau_des]
  Standup with human torque/1 -> "Balancing Controller "/36(STANDUP_WITH_HUMAN_TORQUE)
  human_DoF/1 -> "Balancing Controller "/3(HUMAN_DOF_FOR_SIMULINK)
  "human_w_H_b "/1 -> "Balancing Controller "/37(human_w_H_b)
  "human_qj "/1 -> "Balancing Controller "/38(human_qj)
  human_nu_b/1 -> "Balancing Controller "/39(human_nu_b)
  human_dqj/1 -> "Balancing Controller "/40(human_dqj)
  human_M/1 -> "Balancing Controller "/41(human_M)
  human_bias_torques/1 -> "Balancing Controller "/42(human_h)
  human_torques/1 -> "Balancing Controller "/43(human_torques)
  human_w_H_lFoot/1 -> "Balancing Controller "/44(human_w_H_l_contact)
  human_w_H_rFoot/1 -> "Balancing Controller "/45(human_w_H_r_contact)
  human_JlFoot/1 -> "Balancing Controller "/46(human_JL)
  human_JrFoot/1 -> "Balancing Controller "/47(human_JR)
  human_dJlFootnu/1 -> "Balancing Controller "/48(human_dJL_nu)
  human_dJrFootnu/1 -> "Balancing Controller "/49(human_dJR_nu)
  human_w_H_lArm/1 -> "Balancing Controller "/50(human_w_H_lArm_contact)
  human_w_H_rArm/1 -> "Balancing Controller "/51(human_w_H_rArm_contact)
  human_JlArm/1 -> "Balancing Controller "/52(human_JLArm)
  human_JrArm/1 -> "Balancing Controller "/53(human_JRArm)
  human_dJlArmnu/1 -> "Balancing Controller "/54(human_dJLArm_nu)
  human_dJrArmnu/1 -> "Balancing Controller "/55(human_dJRArm_nu)
  Get Measurement/1 -> "Balancing Controller "/57(robot_torques)
  "Balancing Controller "/19(fArms) -> fArms/1, [fArms]
  "Balancing Controller "/18(alpha) -> [alpha]
  "Balancing Controller "/20(phri_human_feet_wrench) -> [phri_human_feet_wrench]
  "Balancing Controller "/21(phri_robot_feet_wrench) -> [phri_robot_feet_wrench]
  JLArm/1 -> "Balancing Controller "/28(JLArm)
  JRArm/1 -> "Balancing Controller "/29(JRArm)
  dJLArmnu/1 -> "Balancing Controller "/30(dJLArm_nu)
  dJRArmnu/1 -> "Balancing Controller "/31(dJRArm_nu)
  Measured FT/1 -> "Balancing Controller "/35(MEASURED_FT)
  CMM/1 -> "Balancing Controller "/22(CMM)
  "Balancing Controller "/22(correctionFromSupportTorque) -> [corrFromSupportTorque]

== system torqueBalancingPHRIStandup/Robot system/emergency stop: joint limits ==
  qj   EMERGENCY STOP : Inport
  Enable : EnablePort
  Assertion : Assertion
  Get Limits : WBToolboxLibrary/wholeBodyStates/Get Limits  limitsSource=ControlBoard  limitsType=Position
      settings: SourceProductName=Whole Body Toolbox
  MATLAB Function : MATLAB Function  TreatAsAtomicUnit=on
  index1 : Constant  Value=0.01  VectorParams1D=off
  wires:
  Get Limits/1 -> MATLAB Function/1(umin)
  Get Limits/2 -> MATLAB Function/2(umax)
  index1/1 -> MATLAB Function/4(tol)
  qj   EMERGENCY STOP/1 -> MATLAB Function/3(u)
  MATLAB Function/1(inRange) -> Assertion/1

== system torqueBalancingPHRIStandup/Robot system/robot world to human feet transformation ==
  w_H_b : Inport
  qj : Inport  Port=2
  Display{1..4} (4 alike) : Display
  Forward Kinematics : WBToolboxLibrary/wholeBodyModel/Kinematics/Forward Kinematics  frameName=Frames.LEFT_FOOT
      settings: SourceProductName=Whole Body Toolbox
  Forward Kinematics1 : WBToolboxLibrary/wholeBodyModel/Kinematics/Forward Kinematics  frameName=Frames.RIGHT_FOOT
      settings: SourceProductName=Whole Body Toolbox
  MATLAB Function : MATLAB Function  TreatAsAtomicUnit=on
  w_H_humanLeftFeet : Outport
  w_H_humanRightFeet : Outport  Port=2
  wires:
  MATLAB Function/1(w_H_humanLeftFeet) -> w_H_humanLeftFeet/1
  Forward Kinematics1/1 -> Display4/1, MATLAB Function/2(w_H_robotRightFeet)
  Forward Kinematics/1 -> Display2/1, MATLAB Function/1(w_H_robotLeftFeet)
  qj/1 -> Display3/1, Forward Kinematics1/2, Forward Kinematics/2
  w_H_b/1 -> Display1/1, Forward Kinematics1/1, Forward Kinematics/1
  MATLAB Function/2(w_H_humanRightFeet) -> w_H_humanRightFeet/1

== system torqueBalancingPHRIStandup/Robot system/synchronizer ==
  GAZEBO_SYNCHRONIZER : Subsystem
  Logical Operator : Logic  Operator=NOT  AllPortsSameDT=off  OutDataTypeStr=boolean
  "ON_GAZEBO " : Constant  Value=Config.ON_GAZEBO
  REAL_TIME_SYNC : Subsystem
  To Workspace : ToWorkspace  VariableName=yarp_time  SaveFormat=Structure With Time  SampleTime=-1
  Yarp Clock : WBToolboxLibrary/Utilities/Yarp Clock
      settings: SourceProductName=Whole Body Toolbox
  wires:
  Logical Operator/1 -> REAL_TIME_SYNC/Enable
  "ON_GAZEBO "/1 -> GAZEBO_SYNCHRONIZER/Enable, Logical Operator/1
  Yarp Clock/1 -> To Workspace/1

== system torqueBalancingPHRIStandup/Human system/Contact Kinematics/Arm Contact Kinematics ==
  w_H_b : Inport
  qj : Inport  Port=2
  nu_b : Inport  Port=3
  qjdot : Inport  Port=4
  DotJ Nu : WBToolboxLibrary/wholeBodyModel/Jacobians/DotJ Nu  frameName=HUMAN_Frames.LEFT_HAND
      settings: SourceProductName=Whole Body Toolbox
  DotJ Nu1 : WBToolboxLibrary/wholeBodyModel/Jacobians/DotJ Nu  frameName=HUMAN_Frames.RIGHT_HAND
      settings: SourceProductName=Whole Body Toolbox
  Forward Kinematics : WBToolboxLibrary/wholeBodyModel/Kinematics/Forward Kinematics  frameName=HUMAN_Frames.LEFT_HAND
      settings: SourceProductName=Whole Body Toolbox
  Forward Kinematics1 : WBToolboxLibrary/wholeBodyModel/Kinematics/Forward Kinematics  frameName=HUMAN_Frames.RIGHT_HAND
      settings: SourceProductName=Whole Body Toolbox
  Jacobian : WBToolboxLibrary/wholeBodyModel/Jacobians/Jacobian  frameName=HUMAN_Frames.RIGHT_HAND
      settings: SourceProductName=Whole Body Toolbox
  Jacobian1 : WBToolboxLibrary/wholeBodyModel/Jacobians/Jacobian  frameName=HUMAN_Frames.LEFT_HAND
      settings: SourceProductName=Whole Body Toolbox
  w_H_lArm : Outport
  w_H_rArm : Outport  Port=2
  JLArm : Outport  Port=3
  JRArm : Outport  Port=4
  dJLArmnu : Outport  Port=5
  dJRArmnu : Outport  Port=6
  wires:
  Forward Kinematics/1 -> w_H_lArm/1
  Jacobian1/1 -> JLArm/1
  qjdot/1 -> DotJ Nu/4, DotJ Nu1/4
  w_H_b/1 -> Forward Kinematics/1, Jacobian/1, DotJ Nu1/1, DotJ Nu/1, Jacobian1/1, Forward Kinematics1/1
  qj/1 -> DotJ Nu1/2, DotJ Nu/2, Jacobian/2, Jacobian1/2, Forward Kinematics1/2, Forward Kinematics/2
  nu_b/1 -> DotJ Nu/3, DotJ Nu1/3
  Forward Kinematics1/1 -> w_H_rArm/1
  Jacobian/1 -> JRArm/1
  DotJ Nu1/1 -> dJRArmnu/1
  DotJ Nu/1 -> dJLArmnu/1

== system torqueBalancingPHRIStandup/Human system/Contact Kinematics/Leg Contact Kinematics ==
  w_H_b : Inport
  qj : Inport  Port=2
  nu_b : Inport  Port=3
  qjdot : Inport  Port=4
  DotJ Nu : WBToolboxLibrary/wholeBodyModel/Jacobians/DotJ Nu  frameName=HUMAN_Frames.LEFT_FOOT
      settings: SourceProductName=Whole Body Toolbox
  DotJ Nu1 : WBToolboxLibrary/wholeBodyModel/Jacobians/DotJ Nu  frameName=HUMAN_Frames.RIGHT_FOOT
      settings: SourceProductName=Whole Body Toolbox
  Forward Kinematics : WBToolboxLibrary/wholeBodyModel/Kinematics/Forward Kinematics  frameName=HUMAN_Frames.LEFT_FOOT
      settings: SourceProductName=Whole Body Toolbox
  Forward Kinematics1 : WBToolboxLibrary/wholeBodyModel/Kinematics/Forward Kinematics  frameName=HUMAN_Frames.RIGHT_FOOT
      settings: SourceProductName=Whole Body Toolbox
  Jacobian : WBToolboxLibrary/wholeBodyModel/Jacobians/Jacobian  frameName=HUMAN_Frames.RIGHT_FOOT
      settings: SourceProductName=Whole Body Toolbox
  Jacobian1 : WBToolboxLibrary/wholeBodyModel/Jacobians/Jacobian  frameName=HUMAN_Frames.LEFT_FOOT
      settings: SourceProductName=Whole Body Toolbox
  w_H_lFoot : Outport
  w_H_rFoot : Outport  Port=2
  JLFoot : Outport  Port=3
  JRFoot : Outport  Port=4
  dJLFootnu : Outport  Port=5
  dJRFootnu : Outport  Port=6
  wires:
  DotJ Nu/1 -> dJLFootnu/1
  DotJ Nu1/1 -> dJRFootnu/1
  Jacobian/1 -> JRFoot/1
  Forward Kinematics1/1 -> w_H_rFoot/1
  nu_b/1 -> DotJ Nu1/3, DotJ Nu/3
  qj/1 -> Forward Kinematics/2, Forward Kinematics1/2, Jacobian1/2, Jacobian/2, DotJ Nu/2, DotJ Nu1/2
  w_H_b/1 -> Forward Kinematics1/1, Jacobian1/1, DotJ Nu/1, DotJ Nu1/1, Jacobian/1, Forward Kinematics/1
  qjdot/1 -> DotJ Nu1/4, DotJ Nu/4
  Jacobian1/1 -> JLFoot/1
  Forward Kinematics/1 -> w_H_lFoot/1

== system torqueBalancingPHRIStandup/Human system/Dump and visualize/Human data ==
  human_w_H_b : Inport
  human_jointData : Inport  Port=2
  human_jointVelocitiesData : Inport  Port=3
  human_jointTorquesData : Inport  Port=4
  Enable : EnablePort
  " Using Robot Model" : Subsystem
  NOT : Logic  Operator=NOT  IconShape=distinctive  AllPortsSameDT=off  OutDataTypeStr=boolean
  ON_GAZEBO 3 : Constant  Value=Config.USING_HUMAN_MODEL
  Selector : Selector  NumberOfDimensions=2  InputPortWidth=3  IndexOptions=Index vector (dialog),Index vector (dialog)  Indices=[1 2 3],[1 2 3]  OutputSizes=1,1
  Selector1 : Selector  NumberOfDimensions=2  InputPortWidth=3  IndexOptions=Index vector (dialog),Index vector (dialog)  Indices=[1 2 3],4  OutputSizes=1,1
  Using Human Model : Subsystem  Commented=on
  base Pose : Scope  NumInputPorts=2
  wires:
  human_jointData/1 -> Using Human Model/1(human_jointData), " Using Robot Model"/1(human_jointData)
  human_jointVelocitiesData/1 -> Using Human Model/2(human_jointVelocitiesData), " Using Robot Model"/2(human_jointVelocitiesData)
  human_jointTorquesData/1 -> Using Human Model/3(human_jointTorquesData), " Using Robot Model"/3(human_jointTorquesData)
  ON_GAZEBO 3/1 -> Using Human Model/Enable, NOT/1
  Selector/1 -> base Pose/2  "baseOrientation"
  human_w_H_b/1 -> Selector1/1, Selector/1
  Selector1/1 -> base Pose/1  "basePosition"
  NOT/1 -> " Using Robot Model"/Enable

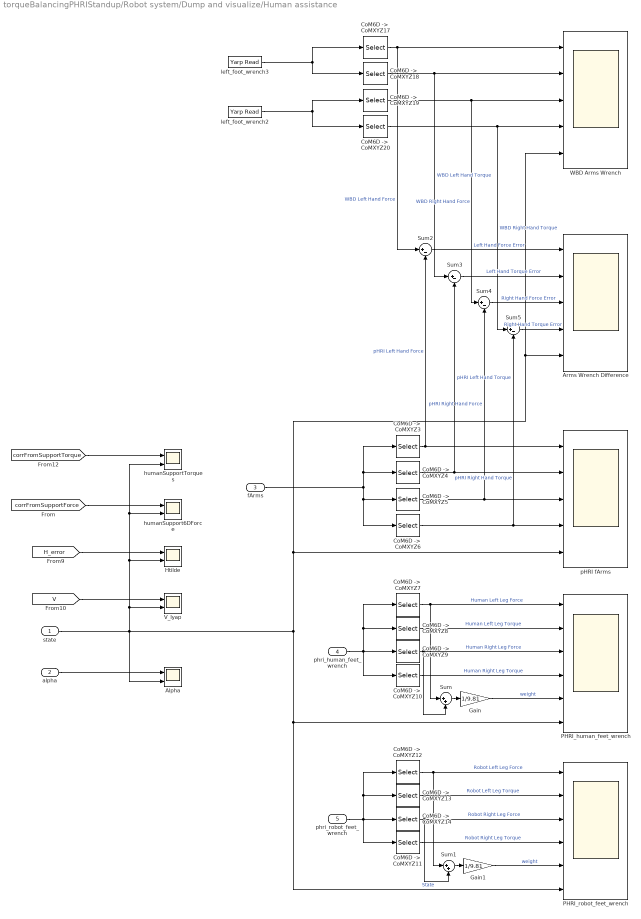
== system torqueBalancingPHRIStandup/Robot system/Dump and visualize/Human assistance ==
  state : Inport
  alpha : Inport  Port=2
  fArms : Inport  Port=3
  phri_human_feet_wrench : Inport  Port=4
  phri_robot_feet_wrench : Inport  Port=5
  Alpha : Scope  NumInputPorts=2
  Arms Wrench Difference : Scope  NumInputPorts=5
  "CoM6D ->  CoMXYZ10" : Selector  InputPortWidth=12  IndexOptions=Index vector (dialog)  Indices=[10 11 12]  OutputSizes=1
  "CoM6D ->  CoMXYZ11" : Selector  InputPortWidth=12  IndexOptions=Index vector (dialog)  Indices=[10 11 12]  OutputSizes=1
  "CoM6D ->  CoMXYZ12" : Selector  InputPortWidth=12  IndexOptions=Index vector (dialog)  Indices=[1 2 3]  OutputSizes=1
  "CoM6D ->  CoMXYZ13" : Selector  InputPortWidth=12  IndexOptions=Index vector (dialog)  Indices=[4 5 6]  OutputSizes=1
  "CoM6D ->  CoMXYZ14" : Selector  InputPortWidth=12  IndexOptions=Index vector (dialog)  Indices=[7 8 9]  OutputSizes=1
  "CoM6D ->  CoMXYZ17" : Selector  InputPortWidth=6  IndexOptions=Index vector (dialog)  Indices=[1 2 3]  OutputSizes=1
  "CoM6D ->  CoMXYZ18" : Selector  InputPortWidth=6  IndexOptions=Index vector (dialog)  Indices=[4 5 6]  OutputSizes=1
  "CoM6D ->  CoMXYZ19" : Selector  InputPortWidth=6  IndexOptions=Index vector (dialog)  Indices=[1 2 3]  OutputSizes=1
  "CoM6D ->  CoMXYZ20" : Selector  InputPortWidth=6  IndexOptions=Index vector (dialog)  Indices=[4 5 6]  OutputSizes=1
  "CoM6D ->  CoMXYZ3" : Selector  InputPortWidth=12  IndexOptions=Index vector (dialog)  Indices=[1 2 3]  OutputSizes=1
  "CoM6D ->  CoMXYZ4" : Selector  InputPortWidth=12  IndexOptions=Index vector (dialog)  Indices=[4 5 6]  OutputSizes=1
  "CoM6D ->  CoMXYZ5" : Selector  InputPortWidth=12  IndexOptions=Index vector (dialog)  Indices=[7 8 9]  OutputSizes=1
  "CoM6D ->  CoMXYZ6" : Selector  InputPortWidth=12  IndexOptions=Index vector (dialog)  Indices=[10 11 12]  OutputSizes=1
  "CoM6D ->  CoMXYZ7" : Selector  InputPortWidth=12  IndexOptions=Index vector (dialog)  Indices=[1 2 3]  OutputSizes=1
  "CoM6D ->  CoMXYZ8" : Selector  InputPortWidth=12  IndexOptions=Index vector (dialog)  Indices=[4 5 6]  OutputSizes=1
  "CoM6D ->  CoMXYZ9" : Selector  InputPortWidth=12  IndexOptions=Index vector (dialog)  Indices=[7 8 9]  OutputSizes=1
  Gain : Gain  Gain=1/9.81
  Gain1 : Gain  Gain=1/9.81
  Htilde : Scope  NumInputPorts=2
  PHRI_human_feet_wrench : Scope  NumInputPorts=6
  PHRI_robot_feet_wrench : Scope  NumInputPorts=6
  Sum : Sum  Inputs=|++
  Sum1 : Sum  Inputs=|++
  Sum{2..5} (4 alike) : Sum  Inputs=|+-
  V_lyap : Scope  NumInputPorts=2
  WBD Arms Wrench : Scope  NumInputPorts=5
  humanSupport6DForce : Scope  NumInputPorts=2
  humanSupportTorques : Scope  NumInputPorts=2
  left_foot_wrench2 : WBToolboxLibrary/Utilities/Yarp Read  portName=Ports.RIGHT_ARM  signalSize=6  timeout=0.5  blocking=off  timestamp=off  autoconnect=on  errorOnConnection=on
      settings: SourceProductName=Whole Body Toolbox
  left_foot_wrench3 : WBToolboxLibrary/Utilities/Yarp Read  portName=Ports.LEFT_ARM  signalSize=6  timeout=0.5  blocking=off  timestamp=off  autoconnect=on  errorOnConnection=on
      settings: SourceProductName=Whole Body Toolbox
  pHRI fArms : Scope  NumInputPorts=5
  wires:
  [H_error] -> Htilde/1
  [corrFromSupportForce] -> humanSupport6DForce/1
  [V] -> V_lyap/1
  "CoM6D ->  CoMXYZ12"/1 -> Sum1/1, PHRI_robot_feet_wrench/1  "Robot Left Leg Force"
  alpha/1 -> Alpha/1
  "CoM6D ->  CoMXYZ11"/1 -> PHRI_robot_feet_wrench/4  "Robot Right Leg Torque"
  "CoM6D ->  CoMXYZ3"/1 -> pHRI fArms/1, Sum2/2  "pHRI Left Hand Force"
  "CoM6D ->  CoMXYZ4"/1 -> Sum3/2, pHRI fArms/2  "pHRI Left Hand Torque"
  "CoM6D ->  CoMXYZ14"/1 -> Sum1/2, PHRI_robot_feet_wrench/3  "Robot Right Leg Force"
  phri_robot_feet_wrench/1 -> "CoM6D ->  CoMXYZ11"/1, "CoM6D ->  CoMXYZ14"/1, "CoM6D ->  CoMXYZ12"/1, "CoM6D ->  CoMXYZ13"/1
  "CoM6D ->  CoMXYZ10"/1 -> PHRI_human_feet_wrench/4  "Human Right Leg Torque"
  "CoM6D ->  CoMXYZ7"/1 -> Sum/1, PHRI_human_feet_wrench/1  "Human Left Leg Force"
  phri_human_feet_wrench/1 -> "CoM6D ->  CoMXYZ10"/1, "CoM6D ->  CoMXYZ9"/1, "CoM6D ->  CoMXYZ8"/1, "CoM6D ->  CoMXYZ7"/1
  "CoM6D ->  CoMXYZ8"/1 -> PHRI_human_feet_wrench/2  "Human Left Leg Torque"
  "CoM6D ->  CoMXYZ9"/1 -> Sum/2, PHRI_human_feet_wrench/3  "Human Right Leg Force"
  "CoM6D ->  CoMXYZ6"/1 -> pHRI fArms/4, Sum5/2  "pHRI Right Hand Torque"
  "CoM6D ->  CoMXYZ5"/1 -> Sum4/2, pHRI fArms/3  "pHRI Right Hand Force"
  "CoM6D ->  CoMXYZ13"/1 -> PHRI_robot_feet_wrench/2  "Robot Left Leg Torque"
  Sum/1 -> Gain/1
  Gain/1 -> PHRI_human_feet_wrench/5  "weight"
  Gain1/1 -> PHRI_robot_feet_wrench/5  "weight"
  Sum1/1 -> Gain1/1
  state/1 -> Alpha/2, pHRI fArms/5, WBD Arms Wrench/5, Arms Wrench Difference/5, PHRI_robot_feet_wrench/6, PHRI_human_feet_wrench/6, V_lyap/2, Htilde/2, humanSupportTorques/2, humanSupport6DForce/2  "State"
  fArms/1 -> "CoM6D ->  CoMXYZ6"/1, "CoM6D ->  CoMXYZ5"/1, "CoM6D ->  CoMXYZ4"/1, "CoM6D ->  CoMXYZ3"/1
  Sum2/1 -> Arms Wrench Difference/1  "Left Hand Force Error"
  Sum3/1 -> Arms Wrench Difference/2  "Left Hand Torque Error"
  Sum4/1 -> Arms Wrench Difference/3  "Right Hand Force Error"
  Sum5/1 -> Arms Wrench Difference/4  "Right Hand Torque Error"
  "CoM6D ->  CoMXYZ18"/1 -> Sum3/1, WBD Arms Wrench/2  "WBD Left Hand Torque"
  "CoM6D ->  CoMXYZ17"/1 -> Sum2/1, WBD Arms Wrench/1  "WBD Left Hand Force"
  left_foot_wrench3/1 -> "CoM6D ->  CoMXYZ18"/1, "CoM6D ->  CoMXYZ17"/1
  "CoM6D ->  CoMXYZ19"/1 -> Sum4/1, WBD Arms Wrench/3  "WBD Right Hand Force"
  "CoM6D ->  CoMXYZ20"/1 -> WBD Arms Wrench/4, Sum5/1  "WBD Right Hand Torque"
  left_foot_wrench2/1 -> "CoM6D ->  CoMXYZ20"/1, "CoM6D ->  CoMXYZ19"/1
  [corrFromSupportTorque] -> humanSupportTorques/1

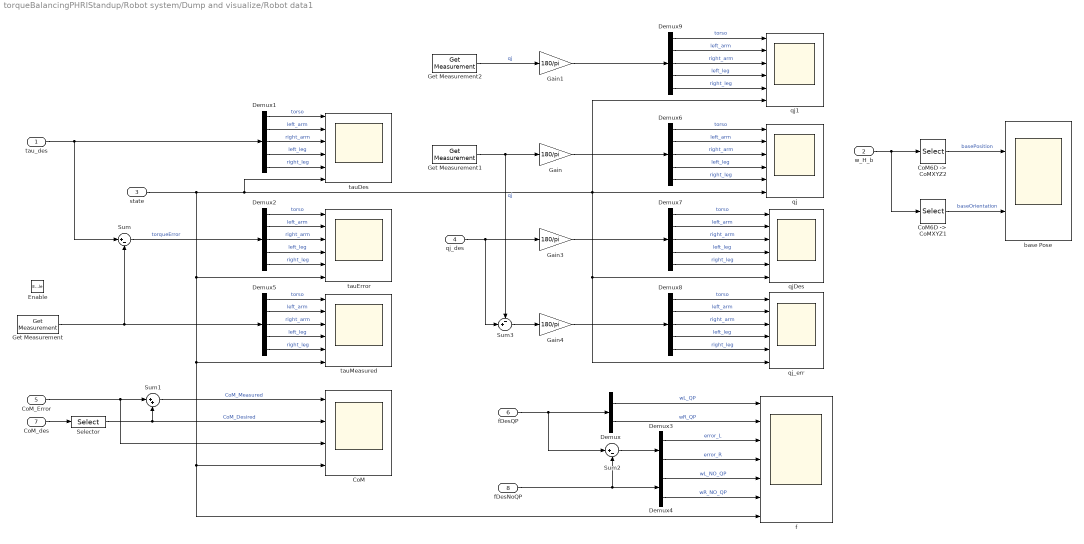
== system torqueBalancingPHRIStandup/Robot system/Dump and visualize/Robot data1 ==
  tau_des : Inport
  w_H_b : Inport  Port=2
  state : Inport  Port=3
  qj_des : Inport  Port=4
  CoM_Error : Inport  Port=5
  fDesQP : Inport  Port=6
  CoM_des : Inport  Port=7
  fDesNoQP : Inport  Port=8
  Enable : EnablePort
  CoM : Scope  NumInputPorts=4
  "CoM6D ->  CoMXYZ1" : Selector  NumberOfDimensions=2  InputPortWidth=7  IndexOptions=Index vector (dialog),Index vector (dialog)  Indices=[1 2 3],[1 2 3]  OutputSizes=1,1
  "CoM6D ->  CoMXYZ2" : Selector  NumberOfDimensions=2  InputPortWidth=7  IndexOptions=Index vector (dialog),Index vector (dialog)  Indices=[1 2 3],[4]  OutputSizes=1,1
  Demux : Demux  Outputs=2
  Demux{1..2,5..9} (7 alike) : Demux  Outputs=Config.numOfJointsForEachControlboard
  Demux3 : Demux  Outputs=2
  Demux4 : Demux  Outputs=2
  Gain{,1,3..4} (4 alike) : Gain  Gain=180/pi
  Get Measurement : WBToolboxLibrary/wholeBodyStates/Get Measurement  measuredType=Joints Torque
      settings: SourceProductName=Whole Body Toolbox
  Get Measurement1 : WBToolboxLibrary/wholeBodyStates/Get Measurement  measuredType=Joints Position
      settings: SourceProductName=Whole Body Toolbox
  Get Measurement2 : WBToolboxLibrary/wholeBodyStates/Get Measurement  measuredType=Joints Velocity
      settings: SourceProductName=Whole Body Toolbox
  Selector : Selector  NumberOfDimensions=2  IndexOptions=Index vector (dialog),Index vector (dialog)  Indices=[1:3],1  OutputSizes=1,1
  Sum : Sum  Inputs=|+-
  Sum1 : Sum  Inputs=|++
  Sum2 : Sum  Inputs=|+-
  Sum3 : Sum  Inputs=-+|
  base Pose : Scope  NumInputPorts=2
  f : Scope  NumInputPorts=7
  qj : Scope  NumInputPorts=6
  qj1 : Scope  NumInputPorts=6
  qjDes : Scope  NumInputPorts=6
  qj_err : Scope  NumInputPorts=6
  tauDes : Scope  NumInputPorts=6
  tauError : Scope  NumInputPorts=6
  tauMeasured : Scope  NumInputPorts=6
  wires:
  CoM_Error/1 -> Sum1/1, CoM/3
  CoM_des/1 -> Selector/1
  Gain/1 -> Demux6/1
  Sum1/1 -> CoM/1  "CoM_Measured"
  Get Measurement1/1 -> Gain/1, Sum3/1  "qj"
  Demux6/5 -> qj/5  "right_leg"
  Demux6/1 -> qj/1  "torso"
  Demux6/2 -> qj/2  "left_arm"
  Demux6/4 -> qj/4  "left_leg"
  fDesQP/1 -> Sum2/1, Demux/1
  Demux6/3 -> qj/3  "right_arm"
  Sum2/1 -> Demux3/1
  fDesNoQP/1 -> Sum2/2, Demux4/1
  tau_des/1 -> Demux1/1, Sum/1
  Get Measurement/1 -> Demux5/1, Sum/2
  Demux1/5 -> tauDes/5  "right_leg"
  Demux1/1 -> tauDes/1  "torso"
  Demux1/2 -> tauDes/2  "left_arm"
  Demux1/4 -> tauDes/4  "left_leg"
  Demux1/3 -> tauDes/3  "right_arm"
  Demux2/5 -> tauError/5  "right_leg"
  Demux2/1 -> tauError/1  "torso"
  Demux2/2 -> tauError/2  "left_arm"
  Demux2/4 -> tauError/4  "left_leg"
  Demux2/3 -> tauError/3  "right_arm"
  Sum/1 -> Demux2/1  "torqueError"
  Demux5/5 -> tauMeasured/5  "right_leg"
  Demux5/1 -> tauMeasured/1  "torso"
  Demux5/2 -> tauMeasured/2  "left_arm"
  Demux5/4 -> tauMeasured/4  "left_leg"
  Demux5/3 -> tauMeasured/3  "right_arm"
  qj_des/1 -> Sum3/2, Gain3/1
  Gain3/1 -> Demux7/1
  Demux7/5 -> qjDes/5  "right_leg"
  Demux7/1 -> qjDes/1  "torso"
  Demux7/2 -> qjDes/2  "left_arm"
  Demux7/4 -> qjDes/4  "left_leg"
  Demux7/3 -> qjDes/3  "right_arm"
  Gain4/1 -> Demux8/1
  Demux8/5 -> qj_err/5  "right_leg"
  Demux8/1 -> qj_err/1  "torso"
  Demux8/2 -> qj_err/2  "left_arm"
  Demux8/4 -> qj_err/4  "left_leg"
  Demux8/3 -> qj_err/3  "right_arm"
  Sum3/1 -> Gain4/1
  Selector/1 -> Sum1/2, CoM/2  "CoM_Desired"
  Demux/1 -> f/1  "wL_QP"
  Demux/2 -> f/2  "wR_QP"
  Demux3/1 -> f/3  "error_L"
  Demux3/2 -> f/4  "error_R"
  Demux4/1 -> f/5  "wL_NO_QP"
  Demux4/2 -> f/6  "wR_NO_QP"
  w_H_b/1 -> "CoM6D ->  CoMXYZ1"/1, "CoM6D ->  CoMXYZ2"/1
  "CoM6D ->  CoMXYZ2"/1 -> base Pose/1  "basePosition"
  "CoM6D ->  CoMXYZ1"/1 -> base Pose/2  "baseOrientation"
  Demux9/5 -> qj1/5  "right_leg"
  Demux9/1 -> qj1/1  "torso"
  Demux9/2 -> qj1/2  "left_arm"
  Get Measurement2/1 -> Gain1/1  "qj"
  Demux9/4 -> qj1/4  "left_leg"
  Demux9/3 -> qj1/3  "right_arm"
  state/1 -> qj1/6, qj_err/6, qjDes/6, qj/6, tauDes/6, f/7, CoM/4, tauMeasured/6, tauError/6
  Gain1/1 -> Demux9/1
